simulink model "UDP_SEND"  (Simulink 8.1)
settings: Solver=ode5  SolverMode=SingleTasking  StartTime=0.0  StopTime=Inf  FixedStep=0.001  RelTol=1e-3
undefined symbols (not defined in the file): generic_ethernet_cb, NumOFWaveforms
libraries: HIL_UDP_lib x9, rtlab x2, simulink x2, opal_lib x1
settings Model: Creator=g73labuser  LastModifiedBy=ed12083  BufferReuse=off
settings DataIOCC: SignalLoggingSaveFormat=Dataset  SaveOutput=off  SaveTime=off
settings OptimizationCC: OptimizeBlockIOStorage=off  BufferReuse=off  ExpressionFolding=off  ExpressionDepthLimit=128  LocalBlockOutputs=off
settings DebuggingCC: FcnCallInpInsideContextMsg=EnableAllAsError  StrictBusMsg=None
settings GRTTargetCC: CombineOutputUpdateFcns=on  GRTInterface=off

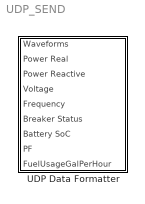
== system UDP_SEND ==
  UDP Data Formatter : Subsystem  mask{ProfileID=1, NumOfWaveforms=3, NumOfPoints=208, NumOfRelays=20, NumOfBatteries=1, NumOfPFs=1, NumOfGensets=2, NumOfMotors=0, NumOfPVs=1}
      mask prompts: ProfileID "Profile ID"; NumOfWaveforms "# of Waveforms"; NumOfPoints "# of Points"; NumOfRelays "# of Relays"; NumOfBatteries "# of Batteries"; NumOfPFs "# of PFs"; NumOfGensets "# of Gensets"; NumOfMotors "# of Motors"; NumOfPVs "# of PVs"

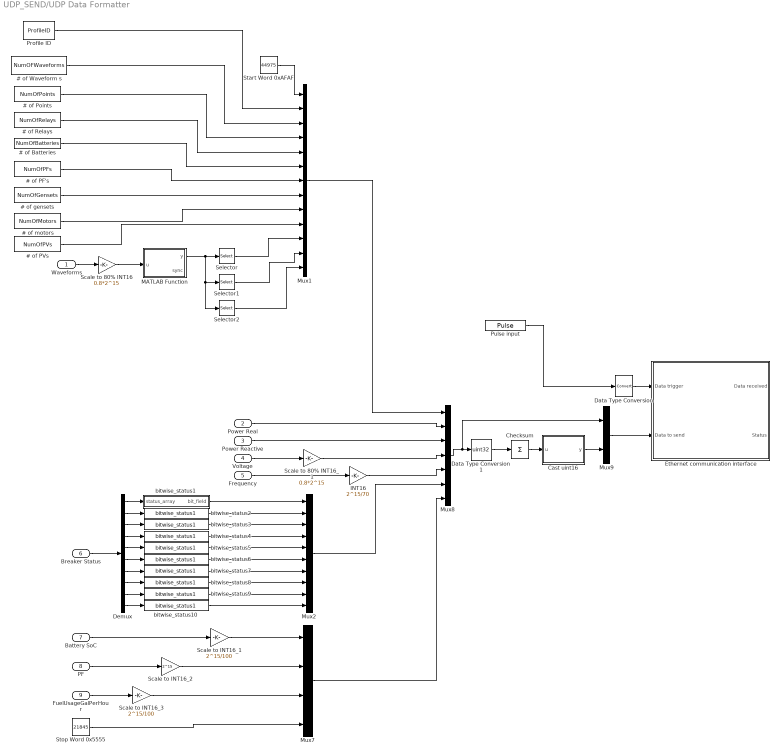
== system UDP_SEND/UDP Data Formatter ==
  Waveforms : Inport  PortDimensions=3
  Power Real : Inport  Port=2  PortDimensions=20
  Power Reactive : Inport  Port=3  PortDimensions=20
  Voltage : Inport  Port=4  PortDimensions=20
  Frequency : Inport  Port=5  PortDimensions=20
  Breaker Status : Inport  Port=6  PortDimensions=20
  Battery SoC : Inport  Port=7  PortDimensions=1
  PF : Inport  Port=8  PortDimensions=1
  FuelUsageGalPerHour : Inport  Port=9  PortDimensions=2
  " # of motors" : Constant  Value=NumOfMotors  OutDataTypeStr=double
  # of Batteries : Constant  Value=NumOfBatteries  OutDataTypeStr=double
  # of PF's : Constant  Value=NumOfPFs  OutDataTypeStr=double
  # of PVs : Constant  Value=NumOfPVs  OutDataTypeStr=double
  # of Points : Constant  Value=NumOfPoints  OutDataTypeStr=double
  # of Relays : Constant  Value=NumOfRelays  OutDataTypeStr=double
  # of Waveform s : Constant  Value=NumOFWaveforms  OutDataTypeStr=double
  # of gensets : Constant  Value=NumOfGensets  OutDataTypeStr=double
  Cast uint16 : MATLAB Function  TreatAsAtomicUnit=on
  Checksum : Sum  Inputs=+
  Data Type Conversion : DataTypeConversion
  Data Type Conversion1 : DataTypeConversion  OutDataTypeStr=uint32  ConvertRealWorld=Stored Integer (SI)  RndMeth=Nearest
  Demux : Demux  Outputs=[2 2 2 2 2 2 2 2 2 2]
  Ethernet communication interface : Subsystem  mask(AsyncEthernet){ctrl_id=1, nbr_to_remote_endpoint=730, type_to_remote_endpoint=INT16, offset_to_remote_endpoint=0, swap_tx=off, nbr_from_remote_endpoint=4, type_from_remote_endpoint=UINT16, offset_from_remote_endpoint=0, swap_rx=off, exe_name='AsyncEthernet', nic_name='eth0', protocol=UDP, tcp_mode=Server, port=7200, remote_ip='255.255.255.255'}
      mask prompts: ctrl_id "Controller ID"; nbr_to_remote_endpoint "Number of data to send"; type_to_remote_endpoint "Type of data to send"; offset_to_remote_endpoint "Byte offset of transmission buffer"; swap_tx "Swap data endianness before transmission"; nbr_from_remote_endpoint "Number of data expected to be received"; type_from_remote_endpoint "Type of data expected to be received"; offset_from_remote_endpoint "Byte offset of reception buffer"; swap_rx "Swap data endianness after reception"; exe_name "Executable name"; nic_name "Network interface name"; tcp_mode "TCP mode"; port "Port number"; remote_ip "Remote IP address"
      mask help: This block is used as a communication interface to send data to a remote dedevice and receive data from it.
      mask Help: eval('rtlab_io_help(''Generic/Ethernet/Ethernet_interface.htm'');');
      mask Callback ctrl_id:
      | var = get_param(gcb,'ctrl_id');
      | set_param([gcb '/AsyncEthernetCtrl'],'ctrl_id',var)
      mask Callback nbr_to_remote_endpoint:
      | var = get_param(gcb,'nbr_to_remote_endpoint');
      | set_param([gcb '/AsyncEthernetCtrl'],'nbr_to_remote_endpoint',var)
      mask TypeOptions type_to_remote_endpoint: UINT8 | INT8 | UINT16 | INT16 | UINT32 | INT32 | FLOAT | DOUBLE
      mask Callback type_to_remote_endpoint:
      | var = get_param(gcb,'type_to_remote_endpoint');
      | set_param([gcb '/AsyncEthernetCtrl'],'type_to_remote_endpoint',var)
      mask Callback offset_to_remote_endpoint:
      | var = get_param(gcb,'offset_to_remote_endpoint');
      | set_param([gcb '/AsyncEthernetCtrl'],'offset_to_remote_endpoint',var)
      mask Callback swap_tx:
      | var = get_param(gcb,'swap_tx');
      | set_param([gcb '/AsyncEthernetCtrl'],'swap_tx',var)
      mask Callback nbr_from_remote_endpoint:
      | var = get_param(gcb,'nbr_from_remote_endpoint');
      | set_param([gcb '/AsyncEthernetCtrl'],'nbr_from_remote_endpoint',var)
      mask TypeOptions type_from_remote_endpoint: UINT8 | INT8 | UINT16 | INT16 | UINT32 | INT32 | FLOAT | DOUBLE
      mask Callback type_from_remote_endpoint:
      | var = get_param(gcb,'type_from_remote_endpoint');
      | set_param([gcb '/AsyncEthernetCtrl'],'type_from_remote_endpoint',var)
      mask Callback offset_from_remote_endpoint:
      | var = get_param(gcb,'offset_from_remote_endpoint');
      | set_param([gcb '/AsyncEthernetCtrl'],'offset_from_remote_endpoint',var)
      mask Callback swap_rx:
      | var = get_param(gcb,'swap_rx');
      | set_param([gcb '/AsyncEthernetCtrl'],'swap_rx',var)
      mask Callback exe_name:
      | str = get_param(gcb,'exe_name');
      | 
      | if exist('str','var')
      |     str = eval(str);
      | end
      | 
      | set_param([gcb '/AsyncEthernetCtrl'],'exe_name',str)
      mask Callback nic_name:
      | str = get_param(gcb,'nic_name');
      | 
      | if exist('str','var')
      |     str = eval(str);
      | end
      | 
      | set_param([gcb '/AsyncEthernetCtrl'],'nic_name',str)
      mask TypeOptions protocol: UDP | TCP
      mask Callback protocol: generic_ethernet_cb('protocol')
      mask TypeOptions tcp_mode: Client | Server
      mask Callback tcp_mode: generic_ethernet_cb('tcp_mode')
      mask Callback port:
      | var = get_param(gcb,'port');
      | set_param([gcb '/AsyncEthernetCtrl'],'port',var)
      mask Callback remote_ip:
      | str = get_param(gcb,'remote_ip');
      | 
      | if exist('str','var')
      |     str = eval(str);
      | end
      | 
      | set_param([gcb '/AsyncEthernetCtrl'],'remote_ip',str)
  INT16 : Gain  Gain=2^15/70
  MATLAB Function : MATLAB Function  TreatAsAtomicUnit=on
  Mux1 : Mux  Inputs=13
  Mux2 : Mux  Inputs=10
  Mux7 : Mux
  Mux8 : Mux  Inputs=7
  Mux9 : Mux  Inputs=2
  Profile ID : Constant  Value=ProfileID  OutDataTypeStr=double
  Pulse input : DiscretePulseGenerator  PulseType=Time based  Period=1/5
  Scale to 80% INT16 : Gain  Gain=0.8*2^15
  Scale to 80% INT16_1 : Gain  Gain=0.8*2^15
  Scale to INT16_1 : Gain  Gain=2^15/100
  Scale to INT16_2 : Gain  Gain=2^15
  Scale to INT16_3 : Gain  Gain=2^15/100
  Selector : Selector  NumberOfDimensions=2  InputPortWidth=3  IndexOptions=Index vector (dialog),Select all  Indices=[1],1  OutputSizes=208,1
  Selector1 : Selector  NumberOfDimensions=2  InputPortWidth=3  IndexOptions=Index vector (dialog),Select all  Indices=[2],1  OutputSizes=208,1
  Selector2 : Selector  NumberOfDimensions=2  InputPortWidth=3  IndexOptions=Index vector (dialog),Select all  Indices=[3],1  OutputSizes=208,1
  Start Word 0xAFAF : Constant  Value=44975  OutDataTypeStr=double
  Stop Word 0x5555 : Constant  Value=21845  OutDataTypeStr=double
  bitwise_status1 : Subsystem
  bitwise_status{2..10} (9 alike) : HIL_UDP_lib/UDP Data Send/bitwise_status1
  wires:
  # of PVs/1 -> Mux1/10
  " # of motors"/1 -> Mux1/9
  # of PF's/1 -> Mux1/7
  # of Batteries/1 -> Mux1/6
  # of gensets/1 -> Mux1/8
  # of Relays/1 -> Mux1/5
  # of Points/1 -> Mux1/4
  # of Waveform s/1 -> Mux1/3
  Profile ID/1 -> Mux1/2
  Start Word 0xAFAF/1 -> Mux1/1
  Pulse input/1 -> Data Type Conversion/1
  Data Type Conversion/1 -> Ethernet communication interface/1(Data trigger)
  Waveforms/1 -> Scale to 80% INT16/1
  MATLAB Function/1(y) -> Selector/1, Selector1/1, Selector2/1
  Selector/1 -> Mux1/11
  Selector1/1 -> Mux1/12
  Selector2/1 -> Mux1/13
  Mux1/1 -> Mux8/1
  Mux8/1 -> Mux9/1, Data Type Conversion1/1
  Checksum/1 -> Cast uint16/1(u)
  Cast uint16/1(y) -> Mux9/2
  Mux9/1 -> Ethernet communication interface/2(Data to send)
  Power Real/1 -> Mux8/2
  Power Reactive/1 -> Mux8/3
  Voltage/1 -> Scale to 80% INT16_1/1
  Frequency/1 -> INT16/1
  Demux/1 -> bitwise_status1/1(status_array)
  Breaker Status/1 -> Demux/1
  Data Type Conversion1/1 -> Checksum/1
  Battery SoC/1 -> Scale to INT16_1/1
  PF/1 -> Scale to INT16_2/1
  Scale to 80% INT16/1 -> MATLAB Function/1(u)
  Scale to 80% INT16_1/1 -> Mux8/4
  INT16/1 -> Mux8/5
  FuelUsageGalPerHour/1 -> Scale to INT16_3/1
  Stop Word 0x5555/1 -> Mux7/4
  Scale to INT16_1/1 -> Mux7/1
  Scale to INT16_2/1 -> Mux7/2
  Scale to INT16_3/1 -> Mux7/3
  Mux2/1 -> Mux8/6
  Mux7/1 -> Mux8/7
  bitwise_status1/1(bit_field) -> Mux2/1
  Demux/2 -> bitwise_status2/1
  Demux/3 -> bitwise_status3/1
  Demux/4 -> bitwise_status4/1
  Demux/5 -> bitwise_status5/1
  Demux/6 -> bitwise_status6/1
  Demux/7 -> bitwise_status7/1
  Demux/8 -> bitwise_status8/1
  Demux/9 -> bitwise_status9/1
  Demux/10 -> bitwise_status10/1
  bitwise_status2/1 -> Mux2/2
  bitwise_status3/1 -> Mux2/3
  bitwise_status4/1 -> Mux2/4
  bitwise_status5/1 -> Mux2/5
  bitwise_status6/1 -> Mux2/6
  bitwise_status7/1 -> Mux2/7
  bitwise_status8/1 -> Mux2/8
  bitwise_status9/1 -> Mux2/9
  bitwise_status10/1 -> Mux2/10

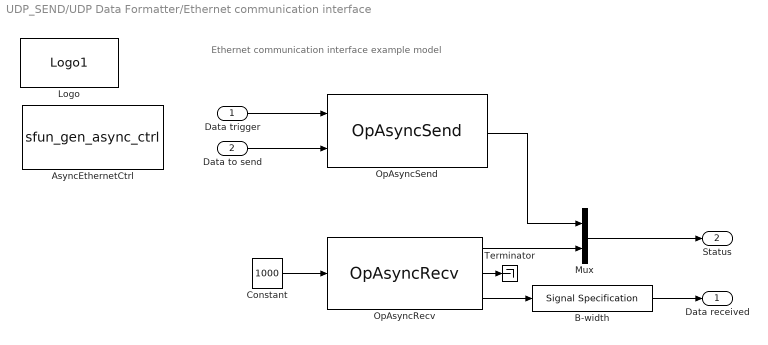
== system UDP_SEND/UDP Data Formatter/Ethernet communication interface ==
  note: Ethernet communication interface example model
  Data trigger : Inport
  Data to send : Inport  Port=2
  AsyncEthernetCtrl : S-Function  InitFcn=generic_ethernet_cb('initfcn');  FunctionName=sfun_gen_async_ctrl  Parameters=ctrl_id, nbr_to_remote_endpoint, type_to_remote_endpoint,nbr_from_remote_endpoint,type_from_remote_endpoint,protocol,tcp_mode, port, offset_to_remote_endpoint,offset_from_remote_endpoint,swap_tx,swap_rx,0,nic_name,remote_ip,'','','','','','','','','','',exe_name,0  EnableBusSupport=off  mask(AsyncEthernetCtrl){ctrl_id=1, nbr_to_remote_endpoint=730, type_to_remote_endpoint=INT16, offset_to_remote_endpoint=0, nbr_from_remote_endpoint=4, type_from_remote_endpoint=UINT16, offset_from_remote_endpoint=0, nic_name=eth0, protocol=UDP, tcp_mode=Server, port=7200, remote_ip=255.255.255.255, exe_name=AsyncEthernet, swap_tx=off, swap_rx=off}
      mask prompts: ctrl_id "Controller ID"; nbr_to_remote_endpoint "Number of data to send"; type_to_remote_endpoint "Type of data to send"; offset_to_remote_endpoint "Byte offset of transmission buffer"; nbr_from_remote_endpoint "Number of data expected to be received"; type_from_remote_endpoint "Type of data expected to be received"; offset_from_remote_endpoint "Byte offset of reception buffer"; nic_name "Network interface name"; tcp_mode "TCP mode"; remote_ip "Remote IP address"; exe_name "Name of the executable"; swap_tx "Swap data endianness before transmission"; swap_rx "Swap data endianness after reception"
      mask help: Generic asynchronous process configuration block
      mask Help: eval('rtlab_help(''opasyncgenctrl'');');
      mask TypeOptions type_to_remote_endpoint: UINT8 | INT8 | UINT16 | INT16 | UINT32 | INT32 | FLOAT | DOUBLE
      mask TypeOptions type_from_remote_endpoint: UINT8 | INT8 | UINT16 | INT16 | UINT32 | INT32 | FLOAT | DOUBLE
      mask TypeOptions protocol: UDP | TCP
      mask TypeOptions tcp_mode: Client | Server
      mask Display: disp(sprintf('\nEthernet communication \ninterface controller\n'))
  B-width : SignalSpecification  Dimensions=nbr_from_remote_endpoint
  Constant : Constant  Value=1000
  Logo : opal_lib/Logo1  vide=[]
  Mux : Mux  Inputs=2
  OpAsyncRecv : rtlab/Communication/Asynchronous/OpAsyncRecv  ctl_id=ctrl_id  recv_id=ctrl_id  enable_param=off  fp1=1  fp2=2  fp3=3  fp4=4  fp5=5  sp1=string1  sp2=string2  sp3=string3  sp4=string4  sp5=string5
  OpAsyncSend : rtlab/Communication/Asynchronous/OpAsyncSend  ctl_id=ctrl_id  send_id=ctrl_id  mode=DONT_NEED_REPLY  enable_param=off  fp1=1  fp2=2  fp3=3  fp4=4  fp5=5  sp1=string1  sp2=string2  sp3=string3  sp4=string4  sp5=string5
  Terminator : Terminator
  Data received : Outport
  Status : Outport  Port=2
  wires:
  B-width/1 -> Data received/1
  OpAsyncRecv/3 -> B-width/1
  OpAsyncRecv/2 -> Terminator/1
  Constant/1 -> OpAsyncRecv/1
  Mux/1 -> Status/1
  OpAsyncRecv/1 -> Mux/2
  OpAsyncSend/1 -> Mux/1
  Data trigger/1 -> OpAsyncSend/1
  Data to send/1 -> OpAsyncSend/2

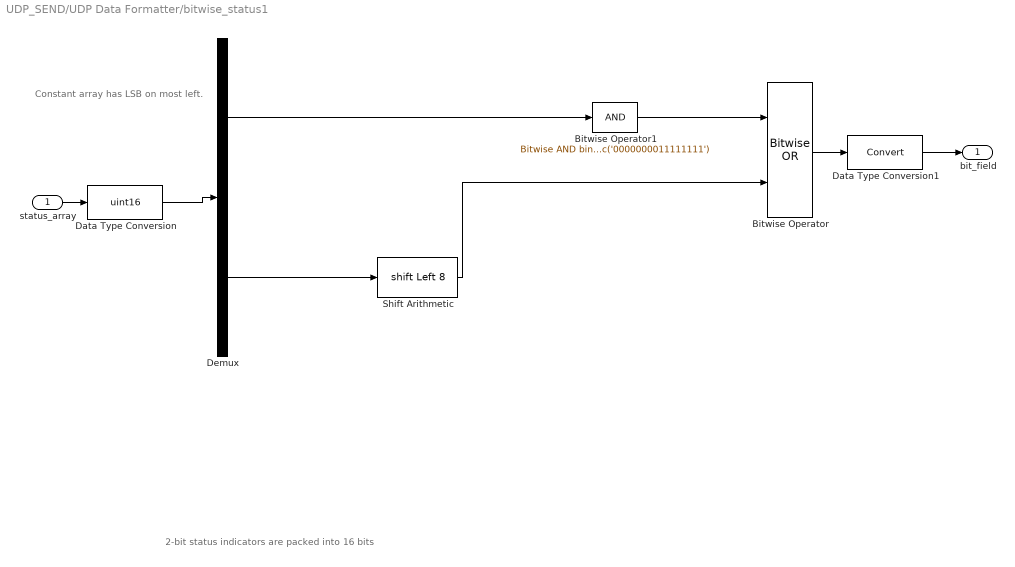
== system UDP_SEND/UDP Data Formatter/bitwise_status1 ==
  note: Constant array has LSB on most left.
  note: 2-bit status indicators are packed into 16 bits
  status_array : Inport
  Bitwise Operator : simulink/Logic and Bit Operations/Bitwise Operator  logicop=OR  UseBitMask=off  NumInputPorts=2  BitMask=bin2dec('11011001')  BitMaskRealWorld=Stored Integer
  Bitwise Operator1 : simulink/Logic and Bit Operations/Bitwise Operator  logicop=AND  UseBitMask=on  BitMask=bin2dec('0000000011111111')  BitMaskRealWorld=Stored Integer
  Data Type Conversion : DataTypeConversion  OutDataTypeStr=uint16
  Data Type Conversion1 : DataTypeConversion
  Demux : Demux  Outputs=2
  Shift Arithmetic : ArithShift  BitShiftNumber=8  BitShiftDirection=Left
  bit_field : Outport
  wires:
  Data Type Conversion1/1 -> bit_field/1
  Bitwise Operator/1 -> Data Type Conversion1/1
  status_array/1 -> Data Type Conversion/1
  Demux/2 -> Shift Arithmetic/1
  Demux/1 -> Bitwise Operator1/1
  Data Type Conversion/1 -> Demux/1
  Shift Arithmetic/1 -> Bitwise Operator/2
  Bitwise Operator1/1 -> Bitwise Operator/1

== matlab function UDP Data Formatter/Cast uint16 ==
  data: u input double; y output double
function y = fcn(u)
%#codegen

x = double(typecast(uint32(u),'uint16'));
y = x(1); % low bits

== matlab function UDP Data Formatter/MATLAB Function ==
  data: u input double; y output double; sync output double
function [y, sync] = fcn(u)
%#codegen

[y, sync] = scopeBuffer(u);
